simulink model "test_Torque_Lagrange1"  (Simulink 10.2)
settings: Solver=ode45  StartTime=0.0  StopTime=2  MaxStep=Step_Time  RelTol=1e-3  EnableMultiTasking=on
settings Model: Creator=saeed  LastModifiedBy=hosse
settings DataIOCC: LimitDataPoints=on
settings OptimizationCC: ExpressionDepthLimit=2147483647
settings DebuggingCC: SaveWithParameterizedLinksMsg=none  SolverPrmCheckMsg=warning  StateNameClashWarn=warning
settings ConfigComp: CovSFcnEnable=off

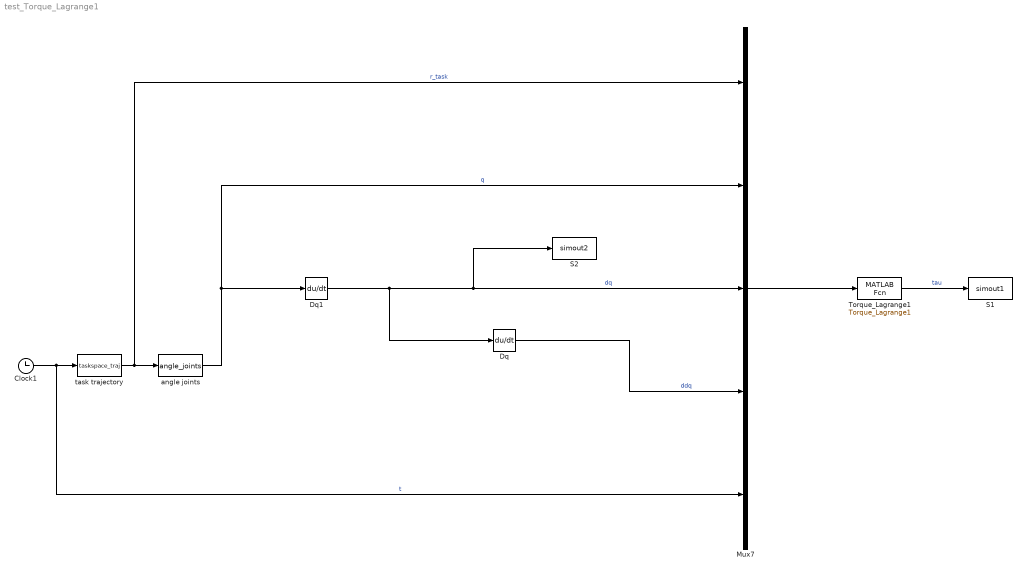
== system test_Torque_Lagrange1 ==
  Clock1 : Clock
  Dq : Derivative
  Dq1 : Derivative
  Mux7 : Mux  Inputs=5
  S1 : ToWorkspace  VariableName=simout1  SaveFormat=Structure With Time  SampleTime=-1
  S2 : ToWorkspace  VariableName=simout2  SaveFormat=Structure With Time  SampleTime=-1
  Torque_Lagrange1 : MATLABFcn  MATLABFcn=Torque_Lagrange1
  angle joints : MATLABFcn  MATLABFcn=angle_joints
  task trajectory : MATLABFcn  MATLABFcn=taskspace_traj
  wires:
  Dq1/1 -> Dq/1, S2/1, Mux7/3  "dq"
  Dq/1 -> Mux7/4  "ddq"
  Torque_Lagrange1/1 -> S1/1  "tau"
  angle joints/1 -> Dq1/1, Mux7/2  "q"
  Mux7/1 -> Torque_Lagrange1/1
  task trajectory/1 -> Mux7/1, angle joints/1  "r_task"
  Clock1/1 -> Mux7/5, task trajectory/1  "t"
